simulink model "MLIinverter"  (R2021a)
settings: Solver=FixedStepAuto  StartTime=0.0  StopTime=1  FixedStep=1e-6  RelTol=1e-3
libraries: spsMosfetLib x24, neural x19, spsTriangleGeneratorLib x12, spsSeriesRLCBranchLib x9, spsSeriesRLCLoadLib x4, spsRMSLib x3, spsVoltageMeasurementLib x3, spsThreePhaseVIMeasurementLib x2, spsNeutralLib x1, spsPVArrayLib x1, simulink x1, spsCurrentMeasurementLib x1
(part 1 of 2)
settings Model: Creator=Administrator  LastModifiedBy=dezir
settings SolverCC: AlgebraicLoopSolver=TrustRegion
settings DebuggingCC: SFMachineParentedDataDiag=warning
settings SFSimCC: CustomCodeUndefinedFunction=UseInterfaceOnly

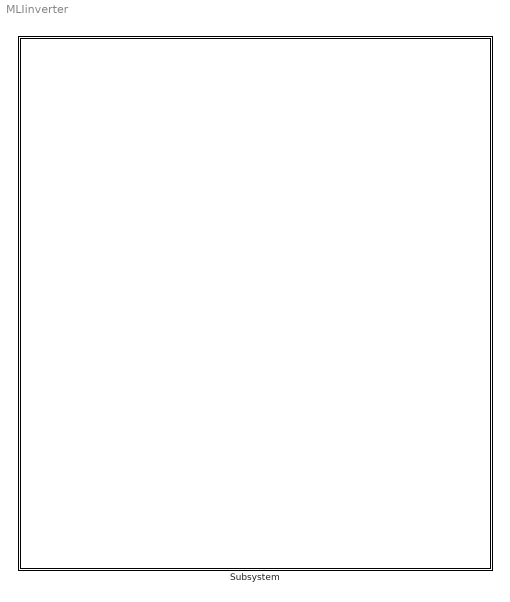
== system MLIinverter ==
  Subsystem : Subsystem

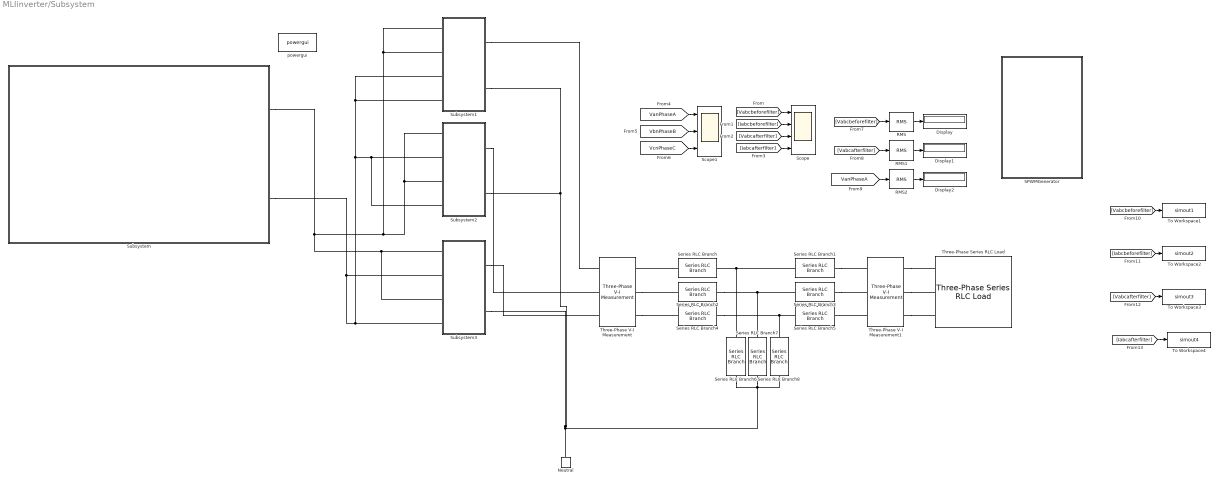
== system MLIinverter/Subsystem ==
  Display : Display
  Display1 : Display
  Display2 : Display
  Neutral : spsNeutralLib/Neutral  LConnTagsString=a  NodeNumber=10
      settings: AttributesFormatString=node %<NodeNumber>  SourceProductBaseCode=PS
  RMS : spsRMSLib/RMS  TrueRMS=on  Freq=50  RMSInit=0  Ts=0
  RMS1 : spsRMSLib/RMS  TrueRMS=on  Freq=50  RMSInit=0  Ts=0
  RMS2 : spsRMSLib/RMS  TrueRMS=on  Freq=50  RMSInit=0  Ts=0
  SPWMGenerator : Subsystem
  Scope : Scope  NumInputPorts=4
  Scope1 : Scope  NumInputPorts=3
  Series RLC Branch : spsSeriesRLCBranchLib/Series RLC Branch  LConnTagsString=__new0  RConnTagsString=__new0  BranchType=L  Resistance=1  Inductance=260e-3  SetiL0=off  InitialCurrent=0  Capacitance=1e-6  Setx0=off  InitialVoltage=0  Measurements=None
  Series RLC Branch1 : spsSeriesRLCBranchLib/Series RLC Branch  LConnTagsString=__new0  RConnTagsString=__new0  BranchType=L  Resistance=1  Inductance=14e-3  SetiL0=off  InitialCurrent=0  Capacitance=1e-6  Setx0=off  InitialVoltage=0  Measurements=None
  Series RLC Branch2 : spsSeriesRLCBranchLib/Series RLC Branch  LConnTagsString=__new0  RConnTagsString=__new0  BranchType=L  Resistance=1  Inductance=260e-3  SetiL0=off  InitialCurrent=0  Capacitance=1e-6  Setx0=off  InitialVoltage=0  Measurements=None
  Series RLC Branch3 : spsSeriesRLCBranchLib/Series RLC Branch  LConnTagsString=__new0  RConnTagsString=__new0  BranchType=L  Resistance=1  Inductance=14e-3  SetiL0=off  InitialCurrent=0  Capacitance=1e-6  Setx0=off  InitialVoltage=0  Measurements=None
  Series RLC Branch4 : spsSeriesRLCBranchLib/Series RLC Branch  LConnTagsString=__new0  RConnTagsString=__new0  BranchType=L  Resistance=1  Inductance=260e-3  SetiL0=off  InitialCurrent=0  Capacitance=1e-6  Setx0=off  InitialVoltage=0  Measurements=None
  Series RLC Branch5 : spsSeriesRLCBranchLib/Series RLC Branch  LConnTagsString=__new0  RConnTagsString=__new0  BranchType=L  Resistance=1  Inductance=14e-3  SetiL0=off  InitialCurrent=0  Capacitance=1e-6  Setx0=off  InitialVoltage=0  Measurements=None
  Series RLC Branch6 : spsSeriesRLCBranchLib/Series RLC Branch  LConnTagsString=__new0  RConnTagsString=__new0  BranchType=C  Resistance=1  Inductance=1e-3  SetiL0=off  InitialCurrent=0  Capacitance=5e-6  Setx0=off  InitialVoltage=0  Measurements=None
  Series RLC Branch7 : spsSeriesRLCBranchLib/Series RLC Branch  LConnTagsString=__new0  RConnTagsString=__new0  BranchType=C  Resistance=1  Inductance=1e-3  SetiL0=off  InitialCurrent=0  Capacitance=5e-6  Setx0=off  InitialVoltage=0  Measurements=None
  Series RLC Branch8 : spsSeriesRLCBranchLib/Series RLC Branch  LConnTagsString=__new0  RConnTagsString=__new0  BranchType=C  Resistance=1  Inductance=1e-3  SetiL0=off  InitialCurrent=0  Capacitance=5e-6  Setx0=off  InitialVoltage=0  Measurements=None
  Subsystem : Subsystem
  Subsystem1 : Subsystem
  Subsystem2 : Subsystem
  Subsystem3 : Subsystem
  Three-Phase Series RLC Load : spsThreePhaseSeriesRLCLoadLib/Three-Phase Series RLC Load  LConnTagsString=A|B|C  Configuration=Y (grounded)  NominalVoltage=400  Vabc=[1e3 1e3 1e3]  Vabcp=[1e3 1e3 1e3]  NominalFrequency=50  UnbalancedPower=off  ActivePower=1e3  InductivePower=0  CapacitivePower=0  Pabc=[10e3 9e3 11e3]  QLabc=[100 90 110]  QCabc=[100 90 110]  Pabcp=[10e3 9e3 11e3]  QLabcp=[100 90 110]  QCabcp=[100 90 110]  Measurements=None  LoadType=constant PQ
  Three-Phase V-I Measurement : spsThreePhaseVIMeasurementLib/Three-Phase V-I Measurement  VoltageMeasurement=phase-to-ground  SetLabelV=on  LabelV=Vabcbeforefilter  Vpu=off  VpuLL=off  CurrentMeasurement=yes  SetLabelI=on  LabelI=Iabcbeforefilter  Ipu=off  Pbase=100e6  Vbase=500e3  OutputType=Complex  PhasorSimulation=off  PSBequivalent=0
  Three-Phase V-I Measurement1 : spsThreePhaseVIMeasurementLib/Three-Phase V-I Measurement  VoltageMeasurement=phase-to-ground  SetLabelV=on  LabelV=Vabcafterfilter  Vpu=off  VpuLL=off  CurrentMeasurement=yes  SetLabelI=on  LabelI=Iabcafterfilter  Ipu=off  Pbase=100e6  Vbase=500e3  OutputType=Complex  PhasorSimulation=off  PSBequivalent=0
  To Workspace1 : ToWorkspace  VariableName=simout1  SaveFormat=Timeseries  SampleTime=-1
  To Workspace2 : ToWorkspace  VariableName=simout2  SaveFormat=Timeseries  SampleTime=-1
  To Workspace3 : ToWorkspace  VariableName=simout3  SaveFormat=Timeseries  SampleTime=-1
  To Workspace4 : ToWorkspace  VariableName=simout4  SaveFormat=Timeseries  SampleTime=-1
  powergui : spspowerguiLib/powergui  Priority=1  SimulationMode=Discrete  SampleTime=6e-6  frequency=60  Iterations=50  frequencyindice=0  Pbase=100e6  ErrMax=1e-4  UnitsV=kV  UnitsW=MW  buscounter=0  FunctionMessages=off  echomessages=off  EnableUseOfTLC=off  CurrentSourceSwitches=off  DisableSnubberDevices=off  DisableRonSwitches=off  DisableVfSwitches=off  DisplayEquations=off  AutomaticDiscreteSolvers=off  SolverType=Tustin/Backward Euler (TBE)  Interpol=off  ExternalGateDelay=off  methode=off  Ts=100  x0status=blocks  SPID=on  SwTol=0  HookPort=off  NonlinearTolerance=0  nMaxIteration=15  ContinueOnMaxIteration=off  RestoreLinks=warning  ResistiveCurrentMeasurement=off  Frange=[0:2:500]  Ylog=off  Xlog=on  ShowGrid=off  save=off  variable=ZData  structure=0  ZoomFFT=off  StartTime=0.0  cycles=1  DisplayStyle=1  fundamental=60  FreqAxis=off  MaxFrequency=1000  frequencyindicesteady=1  RmsSteady=1  display=off
  wires:
  [Iabcbeforefilter] -> Scope/2
  [VcnPhaseC] -> Scope1/3
  [Iabcafterfilter] -> Scope/4
  RMS/1 -> Display/1
  [VanPhaseA] -> Scope1/1
  [VbnPhaseB] -> Scope1/2
  [Vabcbeforefilter] -> Scope/1
  [VanPhaseA] -> RMS2/1
  [Iabcbeforefilter] -> To Workspace2/1
  RMS1/1 -> Display1/1
  [Vabcafterfilter] -> To Workspace3/1
  [Vabcafterfilter] -> RMS1/1
  [Vabcafterfilter] -> Scope/3
  [Iabcafterfilter] -> To Workspace4/1
  RMS2/1 -> Display2/1
  [Vabcbeforefilter] -> RMS/1
  [Vabcbeforefilter] -> To Workspace1/1
  connections:
  Series RLC Branch4/RConn1 -- Series RLC Branch8/LConn1 -- Series RLC Branch5/LConn1
  Series RLC Branch/LConn1 -- Three-Phase V-I Measurement/RConn1
  Three-Phase V-I Measurement/RConn2 -- Series RLC Branch2/LConn1
  Series RLC Branch2/RConn1 -- Series RLC Branch7/LConn1 -- Series RLC Branch3/LConn1
  Series RLC Branch3/RConn1 -- Three-Phase V-I Measurement1/LConn2
  Series RLC Branch1/LConn1 -- Series RLC Branch6/LConn1 -- Series RLC Branch/RConn1
  Three-Phase V-I Measurement1/RConn1 -- Three-Phase Series RLC Load/LConn1
  Subsystem2/RConn2 -- Subsystem1/RConn2 -- Subsystem3/RConn2 -- Neutral/LConn1 -- Series RLC Branch7/RConn1 -- Series RLC Branch6/RConn1 -- Series RLC Branch8/RConn1
  Three-Phase V-I Measurement1/LConn3 -- Series RLC Branch5/RConn1
  Three-Phase V-I Measurement/RConn3 -- Series RLC Branch4/LConn1
  Three-Phase V-I Measurement1/RConn3 -- Three-Phase Series RLC Load/LConn3
  Series RLC Branch1/RConn1 -- Three-Phase V-I Measurement1/LConn1
  Three-Phase V-I Measurement1/RConn2 -- Three-Phase Series RLC Load/LConn2
  Subsystem1/RConn1 -- Three-Phase V-I Measurement/LConn1
  Subsystem/RConn1 -- Subsystem3/LConn3 -- Subsystem3/LConn1 -- Subsystem2/LConn1 -- Subsystem2/LConn3 -- Subsystem1/LConn1 -- Subsystem1/LConn2
  Subsystem/RConn2 -- Subsystem3/LConn4 -- Subsystem2/LConn2 -- Subsystem2/LConn4 -- Subsystem1/LConn4 -- Subsystem1/LConn3 -- Subsystem3/LConn2
  Subsystem2/RConn1 -- Three-Phase V-I Measurement/LConn2
  Subsystem3/RConn1 -- Three-Phase V-I Measurement/LConn3

== system MLIinverter/Subsystem/SPWMGenerator ==
  spwmGen : Subsystem
  spwmGen1 : Subsystem
  spwmGen2 : Subsystem

== system MLIinverter/Subsystem/Subsystem ==
  Custom Neural Network : Subsystem
      mask help: Custom Neural Network
      mask Display: e = 0.06;c1 = [120 150 230]/255;c2 = ([120 150 230]+0)/383;c3 = ([120 150 230]+128)/383;patch([0 1 1 0],[0 0 1 1],c1);patch([0 1 1 1-e 1-e 0+e],[0 0 1 1-e 0+e 0+e],c2);patch([0 0 1 1-e 0+e 0+e],[0 1 1 1-e 1-e 0+e],c3);plot([0 1 1 0 0],[0 0 1 1 0]);fprintf('NNET');port_label('input',1,' Input');port_label('output',1,'Output ');
  PV Array : spsPVArrayLib/PV Array  Npar=20  Nser=10  PlotType=array @ 25 deg.C & specified irradiances  S_vec="[ 1000  500  100 ]"  Temp_C_vec="[ 45 25  ]"  ModuleName=A10Green Technology A10J-M60-240  PlotWhenSelected=off  Pm=240.5376  Ncell=60  Voc=36.84  Isc=8.32  Vm=30.72  Im=7.83  beta_Voc_pc=-0.359  alpha_Isc_pc=0.096995  beta_Voc=-0.13226  alpha_Isc=0.00807  IL=8.3299  I0=2.8736e-10  nI=0.99259  Rsh=330.6558  Rs=0.19366  RobustModel=off  RobustCellTemperature=313.3991  BAL=on  Tc=1e-6  Tfilter=5e-5
  Repeating Sequence : simulink/Sources/Repeating Sequence  rep_seq_t=[0 100]  rep_seq_y=[15 40]
  Subsystem1 : Subsystem
  Subsystem2 : Subsystem
  Uniform Random Number : UniformRandomNumber  Minimum=800  Maximum=1000  SampleTime=0.1
  D : PMIOPort  Side=Right
  S : PMIOPort  Port=2  Side=Right
  tag scope: Irr=global, temp=global
  wires:
  PV Array/1 -> Subsystem1/2(In2)
  Uniform Random Number/1 -> [Irr], PV Array/1
  Repeating Sequence/1 -> [temp], PV Array/2
  Subsystem1/1(Out1) -> Custom Neural Network/1(Input)
  Custom Neural Network/1(Output) -> Subsystem1/1(In1)
  connections:
  Subsystem1/RConn5 -- S/RConn1 -- Subsystem1/RConn4 -- PV Array/RConn2 -- Subsystem1/RConn2 -- Subsystem1/RConn3
  PV Array/RConn1 -- Subsystem1/LConn1
  D/RConn1 -- Subsystem1/RConn1

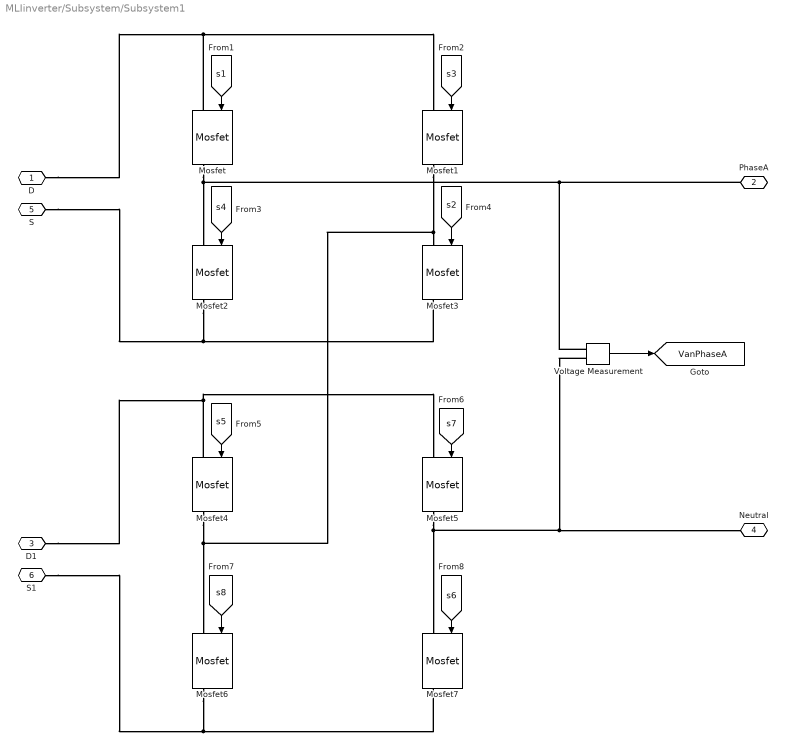
== system MLIinverter/Subsystem/Subsystem1 ==
  Mosfet{,1..7} (8 alike) : spsMosfetLib/Mosfet  Ron=0.1  Lon=0  Rd=0.01  Vfd=0  IC=0  Rs=1e5  Cs=inf  Measurements=on
  Voltage Measurement : spsVoltageMeasurementLib/Voltage Measurement  PhasorSimulation=off  OutputType=Complex  PSBequivalent=0
  D : PMIOPort  Side=Left
  PhaseA : PMIOPort  Port=2  Side=Right
  D1 : PMIOPort  Port=3  Side=Left
  Neutral : PMIOPort  Port=4  Side=Right
  S : PMIOPort  Port=5  Side=Left
  S1 : PMIOPort  Port=6  Side=Left
  tag scope: VanPhaseA=global
  wires:
  [s7] -> Mosfet5/1
  [s4] -> Mosfet2/1
  [s8] -> Mosfet6/1
  [s6] -> Mosfet7/1
  [s2] -> Mosfet3/1
  Voltage Measurement/1 -> [VanPhaseA]
  [s5] -> Mosfet4/1
  [s3] -> Mosfet1/1
  [s1] -> Mosfet/1
  connections:
  Voltage Measurement/LConn1 -- Mosfet/RConn1 -- Mosfet2/LConn1 -- PhaseA/RConn1
  Mosfet/LConn1 -- Mosfet1/LConn1 -- D/RConn1
  D1/RConn1 -- Mosfet4/LConn1 -- Mosfet5/LConn1
  Voltage Measurement/LConn2 -- Mosfet5/RConn1 -- Mosfet7/LConn1 -- Neutral/RConn1
  Mosfet6/RConn1 -- Mosfet7/RConn1 -- S1/RConn1
  Mosfet1/RConn1 -- Mosfet4/RConn1 -- Mosfet6/LConn1 -- Mosfet3/LConn1
  Mosfet2/RConn1 -- Mosfet3/RConn1 -- S/RConn1

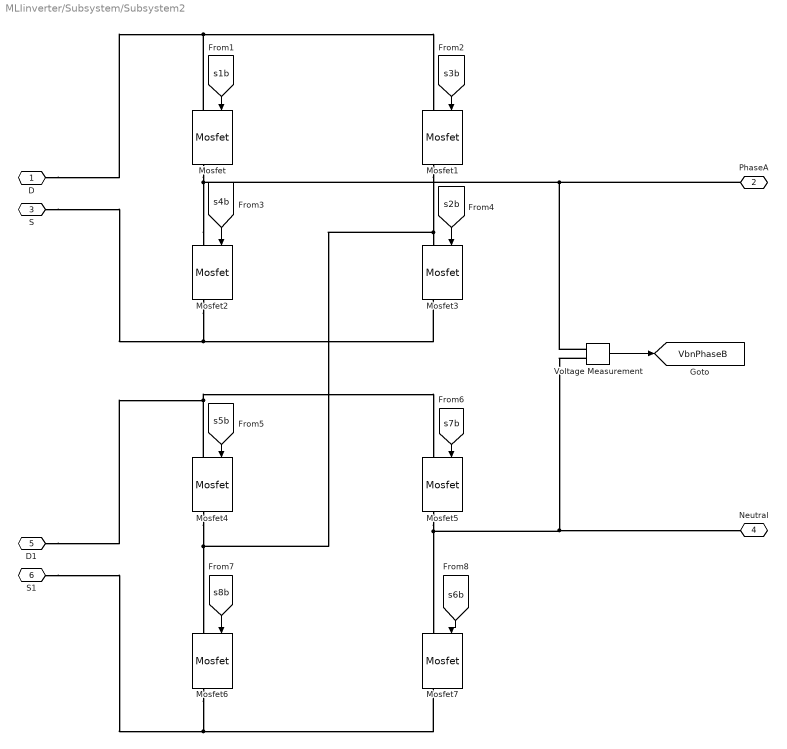
== system MLIinverter/Subsystem/Subsystem2 ==
  Mosfet{,1..7} (8 alike) : spsMosfetLib/Mosfet  Ron=0.1  Lon=0  Rd=0.01  Vfd=0  IC=0  Rs=1e5  Cs=inf  Measurements=on
  Voltage Measurement : spsVoltageMeasurementLib/Voltage Measurement  PhasorSimulation=off  OutputType=Complex  PSBequivalent=0
  D : PMIOPort  Side=Left
  PhaseA : PMIOPort  Port=2  Side=Right
  S : PMIOPort  Port=3  Side=Left
  Neutral : PMIOPort  Port=4  Side=Right
  D1 : PMIOPort  Port=5  Side=Left
  S1 : PMIOPort  Port=6  Side=Left
  tag scope: VbnPhaseB=global
  wires:
  [s7b] -> Mosfet5/1
  [s8b] -> Mosfet6/1
  [s5b] -> Mosfet4/1
  [s2b] -> Mosfet3/1
  [s3b] -> Mosfet1/1
  [s6b] -> Mosfet7/1
  [s1b] -> Mosfet/1
  [s4b] -> Mosfet2/1
  Voltage Measurement/1 -> [VbnPhaseB]
  connections:
  Voltage Measurement/LConn2 -- Mosfet7/LConn1 -- Mosfet5/RConn1 -- Neutral/RConn1
  D1/RConn1 -- Mosfet4/LConn1 -- Mosfet5/LConn1
  Mosfet/LConn1 -- Mosfet1/LConn1 -- D/RConn1
  Mosfet1/RConn1 -- Mosfet6/LConn1 -- Mosfet4/RConn1 -- Mosfet3/LConn1
  Mosfet7/RConn1 -- Mosfet6/RConn1 -- S1/RConn1
  Mosfet2/RConn1 -- Mosfet3/RConn1 -- S/RConn1
  Mosfet2/LConn1 -- Mosfet/RConn1 -- Voltage Measurement/LConn1 -- PhaseA/RConn1

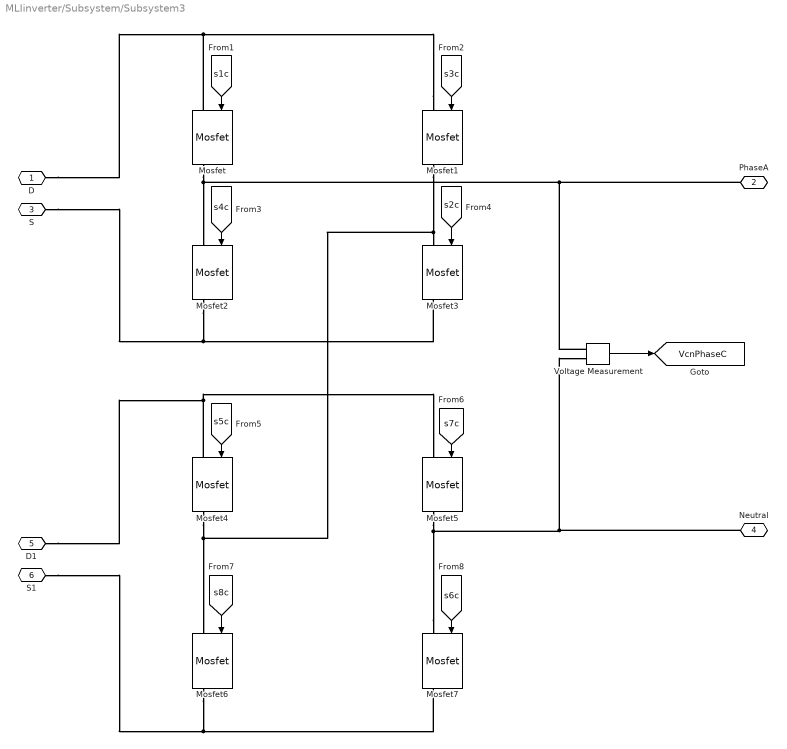
== system MLIinverter/Subsystem/Subsystem3 ==
  Mosfet{,1..7} (8 alike) : spsMosfetLib/Mosfet  Ron=0.1  Lon=0  Rd=0.01  Vfd=0  IC=0  Rs=1e5  Cs=inf  Measurements=on
  Voltage Measurement : spsVoltageMeasurementLib/Voltage Measurement  PhasorSimulation=off  OutputType=Complex  PSBequivalent=0
  D : PMIOPort  Side=Left
  PhaseA : PMIOPort  Port=2  Side=Right
  S : PMIOPort  Port=3  Side=Left
  Neutral : PMIOPort  Port=4  Side=Right
  D1 : PMIOPort  Port=5  Side=Left
  S1 : PMIOPort  Port=6  Side=Left
  tag scope: VcnPhaseC=global
  wires:
  [s2c] -> Mosfet3/1
  [s4c] -> Mosfet2/1
  [s6c] -> Mosfet7/1
  [s1c] -> Mosfet/1
  [s3c] -> Mosfet1/1
  Voltage Measurement/1 -> [VcnPhaseC]
  [s7c] -> Mosfet5/1
  [s8c] -> Mosfet6/1
  [s5c] -> Mosfet4/1
  connections:
  Mosfet6/RConn1 -- Mosfet7/RConn1 -- S1/RConn1
  Voltage Measurement/LConn1 -- Mosfet/RConn1 -- Mosfet2/LConn1 -- PhaseA/RConn1
  Mosfet7/LConn1 -- Mosfet5/RConn1 -- Voltage Measurement/LConn2 -- Neutral/RConn1
  Mosfet1/LConn1 -- Mosfet/LConn1 -- D/RConn1
  D1/RConn1 -- Mosfet4/LConn1 -- Mosfet5/LConn1
  Mosfet1/RConn1 -- Mosfet6/LConn1 -- Mosfet4/RConn1 -- Mosfet3/LConn1
  Mosfet3/RConn1 -- Mosfet2/RConn1 -- S/RConn1

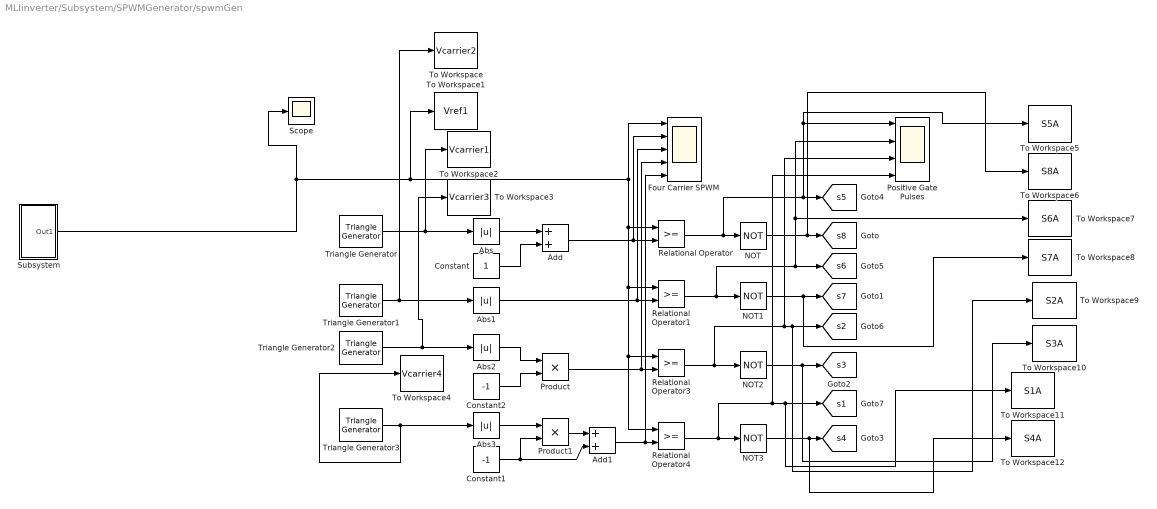
== system MLIinverter/Subsystem/SPWMGenerator/spwmGen ==
  Abs{,1..3} (4 alike) : Abs
  Add : Sum
  Add1 : Sum
  Constant : Constant
  Constant1 : Constant  Value=-1
  Constant2 : Constant  Value=-1
  Four Carrier SPWM : Scope  NumInputPorts=5
  NOT{,1..3} (4 alike) : Logic  Operator=NOT  IconShape=distinctive  AllPortsSameDT=off  OutDataTypeStr=boolean
  Positive Gate Pulses : Scope  NumInputPorts=4
  Product : Product
  Product1 : Product
  Relational Operator{,1,3..4} (4 alike) : RelationalOperator  OutDataTypeStr=boolean  RndMeth=Simplest
  Scope : Scope
  Subsystem : Subsystem
  To Workspace : ToWorkspace  VariableName=Vcarrier2  SampleTime=-1
      settings: Save2DSignal=2-D array (concatenate along first dimension)
  To Workspace1 : ToWorkspace  VariableName=Vref1  SampleTime=-1
      settings: Save2DSignal=2-D array (concatenate along first dimension)
  To Workspace10 : ToWorkspace  VariableName=S3A  SaveFormat=Timeseries  SampleTime=-1
      settings: Save2DSignal=2-D array (concatenate along first dimension)
  To Workspace11 : ToWorkspace  VariableName=S1A  SaveFormat=Timeseries  SampleTime=-1
      settings: Save2DSignal=2-D array (concatenate along first dimension)
  To Workspace12 : ToWorkspace  VariableName=S4A  SaveFormat=Timeseries  SampleTime=-1
      settings: Save2DSignal=2-D array (concatenate along first dimension)
  To Workspace2 : ToWorkspace  VariableName=Vcarrier1  SampleTime=-1
      settings: Save2DSignal=2-D array (concatenate along first dimension)
  To Workspace3 : ToWorkspace  VariableName=Vcarrier3  SampleTime=-1
      settings: Save2DSignal=2-D array (concatenate along first dimension)
  To Workspace4 : ToWorkspace  VariableName=Vcarrier4  SampleTime=-1
      settings: Save2DSignal=2-D array (concatenate along first dimension)
  To Workspace5 : ToWorkspace  VariableName=S5A  SaveFormat=Timeseries  SampleTime=-1
      settings: Save2DSignal=2-D array (concatenate along first dimension)
  To Workspace6 : ToWorkspace  VariableName=S8A  SaveFormat=Timeseries  SampleTime=-1
      settings: Save2DSignal=2-D array (concatenate along first dimension)
  To Workspace7 : ToWorkspace  VariableName=S6A  SaveFormat=Timeseries  SampleTime=-1
      settings: Save2DSignal=2-D array (concatenate along first dimension)
  To Workspace8 : ToWorkspace  VariableName=S7A  SaveFormat=Timeseries  SampleTime=-1
      settings: Save2DSignal=2-D array (concatenate along first dimension)
  To Workspace9 : ToWorkspace  VariableName=S2A  SaveFormat=Timeseries  SampleTime=-1
      settings: Save2DSignal=2-D array (concatenate along first dimension)
  Triangle Generator : spsTriangleGeneratorLib/Triangle Generator  Freq=10e3  Phase=90  Ts=0
  Triangle Generator1 : spsTriangleGeneratorLib/Triangle Generator  Freq=10e3  Phase=90  Ts=0
  Triangle Generator2 : spsTriangleGeneratorLib/Triangle Generator  Freq=10e3  Phase=0  Ts=0
  Triangle Generator3 : spsTriangleGeneratorLib/Triangle Generator  Freq=10e3  Phase=0  Ts=0
  tag scope: s1=global, s2=global, s3=global, s4=global, s5=global, s6=global, s7=global, s8=global
  wires:
  Product1/1 -> Add1/1
  Add1/1 -> Four Carrier SPWM/5, Relational Operator4/2
  NOT3/1 -> To Workspace12/1, [s4]
  Subsystem/1(Out1) -> Scope/1, To Workspace1/1, Four Carrier SPWM/1, Relational Operator/1, Relational Operator4/1, Relational Operator3/1, Relational Operator1/1
  Triangle Generator/1 -> To Workspace2/1, Abs/1
  Constant1/1 -> Add1/2, Product1/2
  Relational Operator/1 -> To Workspace5/1, Positive Gate Pulses/1, [s5], NOT/1
  Add/1 -> Relational Operator/2, Four Carrier SPWM/2
  NOT/1 -> To Workspace6/1, [s8]
  Abs3/1 -> Product1/1
  Abs/1 -> Add/1
  NOT1/1 -> To Workspace8/1, [s7]
  Relational Operator3/1 -> Positive Gate Pulses/3, To Workspace9/1, [s2], NOT2/1
  Abs1/1 -> Relational Operator1/2, Four Carrier SPWM/3
  NOT2/1 -> To Workspace10/1, [s3]
  Product/1 -> Relational Operator3/2, Four Carrier SPWM/4
  Relational Operator1/1 -> To Workspace7/1, Positive Gate Pulses/2, [s6], NOT1/1
  Relational Operator4/1 -> Positive Gate Pulses/4, To Workspace11/1, [s1], NOT3/1
  Triangle Generator3/1 -> To Workspace4/1, Abs3/1
  Triangle Generator1/1 -> To Workspace/1, Abs1/1
  Constant/1 -> Add/2
  Triangle Generator2/1 -> To Workspace3/1, Abs2/1
  Abs2/1 -> Product/1
  Constant2/1 -> Product/2

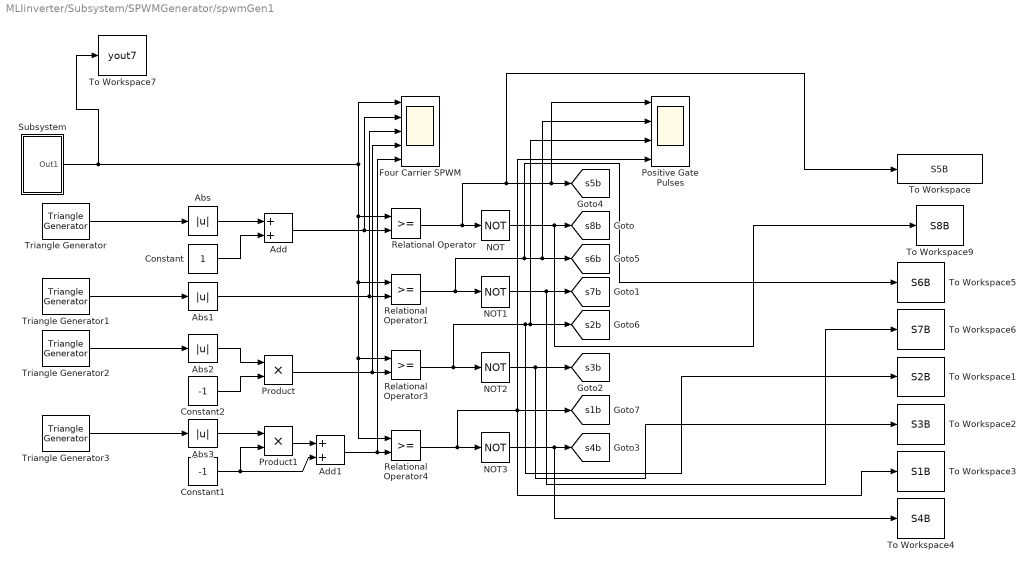
== system MLIinverter/Subsystem/SPWMGenerator/spwmGen1 ==
  Abs{,1..3} (4 alike) : Abs
  Add : Sum
  Add1 : Sum
  Constant : Constant
  Constant1 : Constant  Value=-1
  Constant2 : Constant  Value=-1
  Four Carrier SPWM : Scope  NumInputPorts=5
  NOT{,1..3} (4 alike) : Logic  Operator=NOT  IconShape=distinctive  AllPortsSameDT=off  OutDataTypeStr=boolean
  Positive Gate Pulses : Scope  NumInputPorts=4
  Product : Product
  Product1 : Product
  Relational Operator{,1,3..4} (4 alike) : RelationalOperator  OutDataTypeStr=boolean  RndMeth=Simplest
  Subsystem : Subsystem
  To Workspace : ToWorkspace  VariableName=S5B  SaveFormat=Timeseries  SampleTime=-1
      settings: Save2DSignal=2-D array (concatenate along first dimension)
  To Workspace1 : ToWorkspace  VariableName=S2B  SaveFormat=Timeseries  SampleTime=-1
      settings: Save2DSignal=2-D array (concatenate along first dimension)
  To Workspace2 : ToWorkspace  VariableName=S3B  SaveFormat=Timeseries  SampleTime=-1
      settings: Save2DSignal=2-D array (concatenate along first dimension)
  To Workspace3 : ToWorkspace  VariableName=S1B  SaveFormat=Timeseries  SampleTime=-1
      settings: Save2DSignal=2-D array (concatenate along first dimension)
  To Workspace4 : ToWorkspace  VariableName=S4B  SaveFormat=Timeseries  SampleTime=-1
      settings: Save2DSignal=2-D array (concatenate along first dimension)
  To Workspace5 : ToWorkspace  VariableName=S6B  SaveFormat=Timeseries  SampleTime=-1
      settings: Save2DSignal=2-D array (concatenate along first dimension)
  To Workspace6 : ToWorkspace  VariableName=S7B  SaveFormat=Timeseries  SampleTime=-1
      settings: Save2DSignal=2-D array (concatenate along first dimension)
  To Workspace7 : ToWorkspace  VariableName=yout7  SampleTime=-1
      settings: Save2DSignal=2-D array (concatenate along first dimension)
  To Workspace9 : ToWorkspace  VariableName=S8B  SaveFormat=Timeseries  SampleTime=-1
      settings: Save2DSignal=2-D array (concatenate along first dimension)
  Triangle Generator : spsTriangleGeneratorLib/Triangle Generator  Freq=10e3  Phase=90  Ts=0
  Triangle Generator1 : spsTriangleGeneratorLib/Triangle Generator  Freq=10e3  Phase=90  Ts=0
  Triangle Generator2 : spsTriangleGeneratorLib/Triangle Generator  Freq=10e3  Phase=0  Ts=0
  Triangle Generator3 : spsTriangleGeneratorLib/Triangle Generator  Freq=10e3  Phase=0  Ts=0
  tag scope: s1b=global, s2b=global, s3b=global, s4b=global, s5b=global, s6b=global, s7b=global, s8b=global
  wires:
  Constant2/1 -> Product/2
  Abs2/1 -> Product/1
  Triangle Generator2/1 -> Abs2/1
  Constant/1 -> Add/2
  Triangle Generator1/1 -> Abs1/1
  Triangle Generator3/1 -> Abs3/1
  Relational Operator4/1 -> NOT3/1, To Workspace3/1, [s1b], Positive Gate Pulses/4
  Relational Operator1/1 -> NOT1/1, To Workspace5/1, [s6b], Positive Gate Pulses/2
  Product/1 -> Four Carrier SPWM/4, Relational Operator3/2
  NOT2/1 -> To Workspace2/1, [s3b]
  Abs1/1 -> Four Carrier SPWM/3, Relational Operator1/2
  Relational Operator3/1 -> NOT2/1, To Workspace1/1, [s2b], Positive Gate Pulses/3
  NOT1/1 -> To Workspace6/1, [s7b]
  Abs/1 -> Add/1
  Abs3/1 -> Product1/1
  NOT/1 -> To Workspace9/1, [s8b]
  Add/1 -> Four Carrier SPWM/2, Relational Operator/2
  Relational Operator/1 -> NOT/1, To Workspace/1, [s5b], Positive Gate Pulses/1
  Constant1/1 -> Product1/2, Add1/2
  Triangle Generator/1 -> Abs/1
  Subsystem/1(Out1) -> To Workspace7/1, Relational Operator1/1, Relational Operator3/1, Relational Operator4/1, Relational Operator/1, Four Carrier SPWM/1
  NOT3/1 -> To Workspace4/1, [s4b]
  Add1/1 -> Relational Operator4/2, Four Carrier SPWM/5
  Product1/1 -> Add1/1

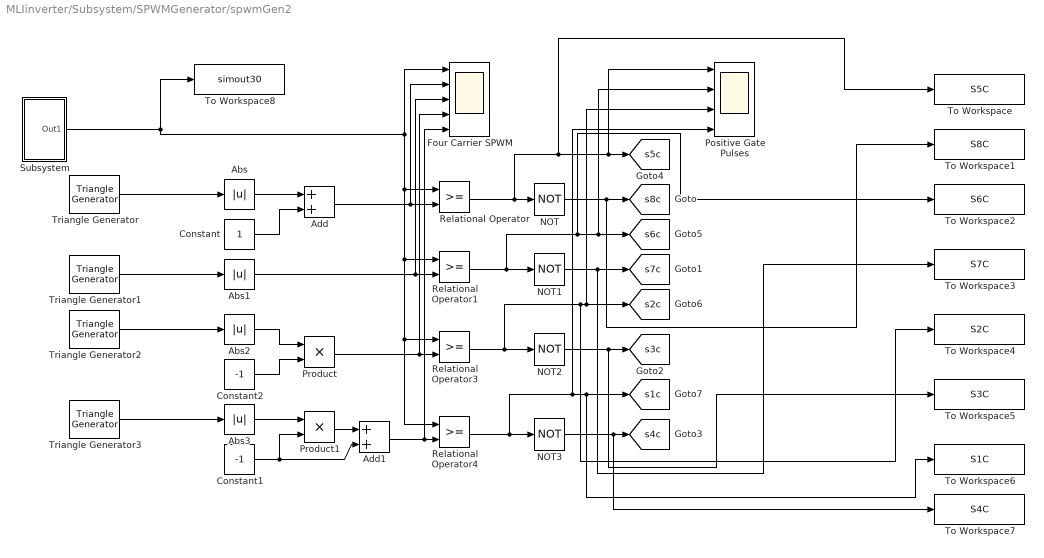
== system MLIinverter/Subsystem/SPWMGenerator/spwmGen2 ==
  Abs{,1..3} (4 alike) : Abs
  Add : Sum
  Add1 : Sum
  Constant : Constant
  Constant1 : Constant  Value=-1
  Constant2 : Constant  Value=-1
  Four Carrier SPWM : Scope  NumInputPorts=5
  NOT{,1..3} (4 alike) : Logic  Operator=NOT  IconShape=distinctive  AllPortsSameDT=off  OutDataTypeStr=boolean
  Positive Gate Pulses : Scope  NumInputPorts=4
  Product : Product
  Product1 : Product
  Relational Operator{,1,3..4} (4 alike) : RelationalOperator  OutDataTypeStr=boolean  RndMeth=Simplest
  Subsystem : Subsystem
  To Workspace : ToWorkspace  VariableName=S5C  SaveFormat=Timeseries  SampleTime=-1
      settings: Save2DSignal=2-D array (concatenate along first dimension)
  To Workspace1 : ToWorkspace  VariableName=S8C  SaveFormat=Timeseries  SampleTime=-1
      settings: Save2DSignal=2-D array (concatenate along first dimension)
  To Workspace2 : ToWorkspace  VariableName=S6C  SaveFormat=Timeseries  SampleTime=-1
      settings: Save2DSignal=2-D array (concatenate along first dimension)
  To Workspace3 : ToWorkspace  VariableName=S7C  SaveFormat=Timeseries  SampleTime=-1
      settings: Save2DSignal=2-D array (concatenate along first dimension)
  To Workspace4 : ToWorkspace  VariableName=S2C  SaveFormat=Timeseries  SampleTime=-1
      settings: Save2DSignal=2-D array (concatenate along first dimension)
  To Workspace5 : ToWorkspace  VariableName=S3C  SaveFormat=Timeseries  SampleTime=-1
      settings: Save2DSignal=2-D array (concatenate along first dimension)
  To Workspace6 : ToWorkspace  VariableName=S1C  SaveFormat=Timeseries  SampleTime=-1
      settings: Save2DSignal=2-D array (concatenate along first dimension)
  To Workspace7 : ToWorkspace  VariableName=S4C  SaveFormat=Timeseries  SampleTime=-1
      settings: Save2DSignal=2-D array (concatenate along first dimension)
  To Workspace8 : ToWorkspace  VariableName=simout30  SampleTime=-1
      settings: Save2DSignal=2-D array (concatenate along first dimension)
  Triangle Generator : spsTriangleGeneratorLib/Triangle Generator  Freq=10e3  Phase=90  Ts=0
  Triangle Generator1 : spsTriangleGeneratorLib/Triangle Generator  Freq=10e3  Phase=90  Ts=0
  Triangle Generator2 : spsTriangleGeneratorLib/Triangle Generator  Freq=10e3  Phase=0  Ts=0
  Triangle Generator3 : spsTriangleGeneratorLib/Triangle Generator  Freq=10e3  Phase=0  Ts=0
  tag scope: s1c=global, s2c=global, s3c=global, s4c=global, s5c=global, s6c=global, s7c=global, s8c=global
  wires:
  Product1/1 -> Add1/1
  Add1/1 -> Four Carrier SPWM/5, Relational Operator4/2
  NOT3/1 -> To Workspace7/1, [s4c]
  Subsystem/1(Out1) -> Four Carrier SPWM/1, Relational Operator/1, Relational Operator4/1, Relational Operator3/1, Relational Operator1/1, To Workspace8/1
  Triangle Generator/1 -> Abs/1
  Constant1/1 -> Add1/2, Product1/2
  Relational Operator/1 -> To Workspace/1, Positive Gate Pulses/1, [s5c], NOT/1
  Add/1 -> Relational Operator/2, Four Carrier SPWM/2
  NOT/1 -> To Workspace1/1, [s8c]
  Abs3/1 -> Product1/1
  Abs/1 -> Add/1
  NOT1/1 -> To Workspace3/1, [s7c]
  Relational Operator3/1 -> To Workspace4/1, Positive Gate Pulses/3, [s2c], NOT2/1
  Abs1/1 -> Relational Operator1/2, Four Carrier SPWM/3
  NOT2/1 -> To Workspace5/1, [s3c]
  Product/1 -> Relational Operator3/2, Four Carrier SPWM/4
  Relational Operator1/1 -> To Workspace2/1, Positive Gate Pulses/2, [s6c], NOT1/1
  Relational Operator4/1 -> Positive Gate Pulses/4, To Workspace6/1, [s1c], NOT3/1
  Triangle Generator3/1 -> Abs3/1
  Triangle Generator1/1 -> Abs1/1
  Constant/1 -> Add/2
  Triangle Generator2/1 -> Abs2/1
  Abs2/1 -> Product/1
  Constant2/1 -> Product/2

== system MLIinverter/Subsystem/Subsystem/Custom Neural Network ==
  Input : Inport  PortDimensions=3
      mask Display: e = 0.06;c1 = [120 230 180]/255;c2 = ([120 230 180]+0)/(256+128);c3 = ([120 230 180]+128)/(256+128);patch([0 1 1 0],[0 0 1 1],c1);patch([0 1 1 1-e 1-e 0+e],[0 0 1 1-e 0+e 0+e],c2);patch([0 0 1 1-e 0+e 0+e],[0 1 1 1-e 1-e 0+e],c3);plot([0 1 1 0 0],[0 0 1 1 0]);
  Layer 1 : Subsystem
      mask Display: e = 0.06;c1 = [120 150 230]/255;c2 = ([120 150 230]+0)/383;c3 = ([120 150 230]+128)/383;patch([0 1 1 0],[0 0 1 1],c1);patch([0 1 1 1-e 1-e 0+e],[0 0 1 1-e 0+e 0+e],c2);patch([0 0 1 1-e 0+e 0+e],[0 1 1 1-e 1-e 0+e],c3);plot([0 1 1 0 0],[0 0 1 1 0]);
  Layer 2 : Subsystem
      mask Display: e = 0.06;c1 = [120 150 230]/255;c2 = ([120 150 230]+0)/383;c3 = ([120 150 230]+128)/383;patch([0 1 1 0],[0 0 1 1],c1);patch([0 1 1 1-e 1-e 0+e],[0 0 1 1-e 0+e 0+e],c2);patch([0 0 1 1-e 0+e 0+e],[0 1 1 1-e 1-e 0+e],c3);plot([0 1 1 0 0],[0 0 1 1 0]);
  Layer 3 : Subsystem
      mask Display: e = 0.06;c1 = [120 150 230]/255;c2 = ([120 150 230]+0)/383;c3 = ([120 150 230]+128)/383;patch([0 1 1 0],[0 0 1 1],c1);patch([0 1 1 1-e 1-e 0+e],[0 0 1 1-e 0+e 0+e],c2);patch([0 0 1 1-e 0+e 0+e],[0 1 1 1-e 1-e 0+e],c3);plot([0 1 1 0 0],[0 0 1 1 0]);
  Process Input 1 : Subsystem
      mask Display: e = 0.06;c1 = [120 150 230]/255;c2 = ([120 150 230]+0)/383;c3 = ([120 150 230]+128)/383;patch([0 1 1 0],[0 0 1 1],c1);patch([0 1 1 1-e 1-e 0+e],[0 0 1 1-e 0+e 0+e],c2);patch([0 0 1 1-e 0+e 0+e],[0 1 1 1-e 1-e 0+e],c3);plot([0 1 1 0 0],[0 0 1 1 0]);
  Process Output 1 : Subsystem
      mask Display: e = 0.06;c1 = [120 150 230]/255;c2 = ([120 150 230]+0)/383;c3 = ([120 150 230]+128)/383;patch([0 1 1 0],[0 0 1 1],c1);patch([0 1 1 1-e 1-e 0+e],[0 0 1 1-e 0+e 0+e],c2);patch([0 0 1 1-e 0+e 0+e],[0 1 1 1-e 1-e 0+e],c3);plot([0 1 1 0 0],[0 0 1 1 0]);
  Output : Outport  InitialOutput=0
      mask Display: e = 0.06;c1 = [120 230 180]/255;c2 = ([120 230 180]+0)/(256+128);c3 = ([120 230 180]+128)/(256+128);patch([0 1 1 0],[0 0 1 1],c1);patch([0 1 1 1-e 1-e 0+e],[0 0 1 1-e 0+e 0+e],c2);patch([0 0 1 1-e 0+e 0+e],[0 1 1 1-e 1-e 0+e],c3);plot([0 1 1 0 0],[0 0 1 1 0]);
  wires:
  Input/1 -> Process Input 1/1(x)
  Process Output 1/1(y) -> Output/1
  Process Input 1/1(p) -> Layer 1/1("p{1}")
  Layer 1/1("a{1}") -> [feedback1]
  [feedback1] -> Layer 2/1("a{1} ")
  Layer 2/1("a{2}") -> [feedback2]
  [feedback2] -> Layer 3/1("a{2} ")
  Layer 3/1("a{3}") -> Process Output 1/1(a)

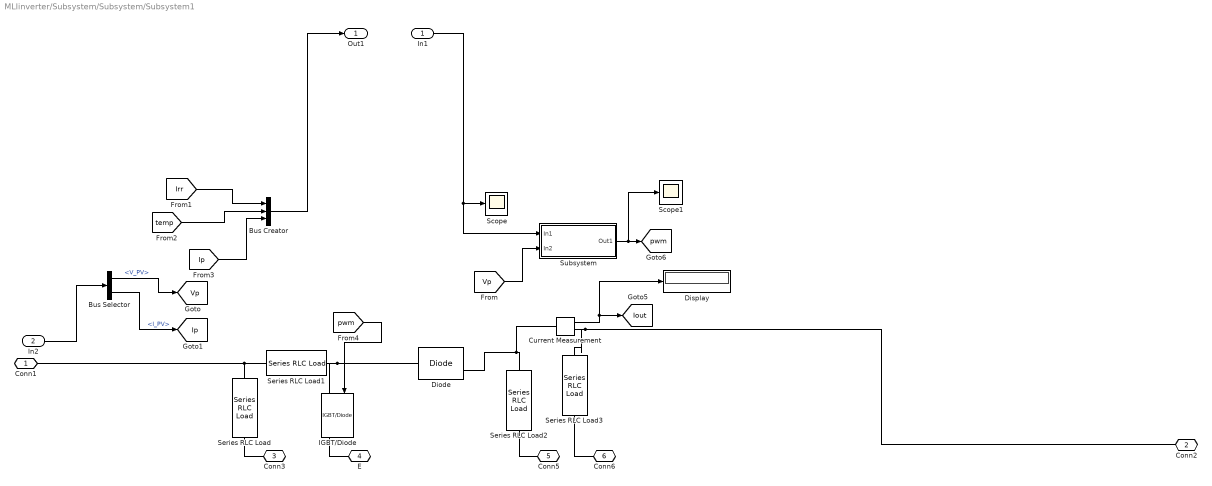
== system MLIinverter/Subsystem/Subsystem/Subsystem1 ==
  In1 : Inport
  In2 : Inport  Port=2
  Bus Creator : BusCreator  Inputs=3
  Bus Selector : BusSelector  OutputSignals=V_PV,I_PV
  Current Measurement : spsCurrentMeasurementLib/Current Measurement  PhasorSimulation=off  OutputType=Complex  PSBequivalent=0
  Diode : spsDiodeLib/Diode  Ron=0.001  Lon=0  Vf=0.8  IC=0  UseSnubber=0  Rs=500  Cs=250e-9  Measurements=on
  Display : Display
  IGBT/Diode : spsIGBTDiodeLib/IGBT//Diode  Ron=1e-3  Rs=1e5  Cs=inf  Measurements=on
  Scope : Scope
  Scope1 : Scope
  Series RLC Load : spsSeriesRLCLoadLib/Series RLC Load  LConnTagsString=a  RConnTagsString=__new0  NominalVoltage=100  NominalFrequency=50  ActivePower=2  InductivePower=0  CapacitivePower=314  Setx0=off  InitialVoltage=0  SetiL0=off  InitialCurrent=0  Measurements=None  LoadType=constant Z
  Series RLC Load1 : spsSeriesRLCLoadLib/Series RLC Load  LConnTagsString=a  RConnTagsString=__new0  NominalVoltage=100  NominalFrequency=50  ActivePower=2  InductivePower=314  CapacitivePower=0  Setx0=off  InitialVoltage=0  SetiL0=off  InitialCurrent=0  Measurements=None  LoadType=constant Z
  Series RLC Load2 : spsSeriesRLCLoadLib/Series RLC Load  LConnTagsString=a  RConnTagsString=__new0  NominalVoltage=100  NominalFrequency=50  ActivePower=2  InductivePower=0  CapacitivePower=314  Setx0=off  InitialVoltage=0  SetiL0=off  InitialCurrent=0  Measurements=None  LoadType=constant Z
  Series RLC Load3 : spsSeriesRLCLoadLib/Series RLC Load  LConnTagsString=a  RConnTagsString=__new0  NominalVoltage=100  NominalFrequency=50  ActivePower=1086.95  InductivePower=0  CapacitivePower=0  Setx0=off  InitialVoltage=0  SetiL0=off  InitialCurrent=0  Measurements=None  LoadType=constant Z
  Subsystem : Subsystem
  Conn1 : PMIOPort  Side=Left
  Conn2 : PMIOPort  Port=2  Side=Right
  Conn3 : PMIOPort  Port=3  Side=Right
  E : PMIOPort  Port=4  Side=Right
  Conn5 : PMIOPort  Port=5  Side=Right
  Conn6 : PMIOPort  Port=6  Side=Right
  Out1 : Outport
  tag scope: Iout=global, Ip=global, Vp=global, pwm=global
  wires:
  In1/1 -> Subsystem/1(In1), Scope/1
  Subsystem/1(Out1) -> Scope1/1, [pwm]
  [temp] -> Bus Creator/2
  [Vp] -> Subsystem/2(In2)
  Bus Selector/2 -> [Ip]  "<I_PV>"
  [pwm] -> IGBT/Diode/1
  [Irr] -> Bus Creator/1
  Bus Selector/1 -> [Vp]  "<V_PV>"
  [Ip] -> Bus Creator/3
  Current Measurement/1 -> Display/1, [Iout]
  In2/1 -> Bus Selector/1
  Bus Creator/1 -> Out1/1
  connections:
  Series RLC Load1/RConn1 -- IGBT/Diode/LConn1 -- Diode/LConn1
  Series RLC Load/LConn1 -- Series RLC Load1/LConn1 -- Conn1/RConn1
  Series RLC Load2/RConn1 -- Conn5/RConn1
  IGBT/Diode/RConn1 -- E/RConn1
  Diode/RConn1 -- Current Measurement/LConn1 -- Series RLC Load2/LConn1
  Current Measurement/RConn1 -- Series RLC Load3/LConn1 -- Conn2/RConn1
  Series RLC Load3/RConn1 -- Conn6/RConn1
  Conn3/RConn1 -- Series RLC Load/RConn1

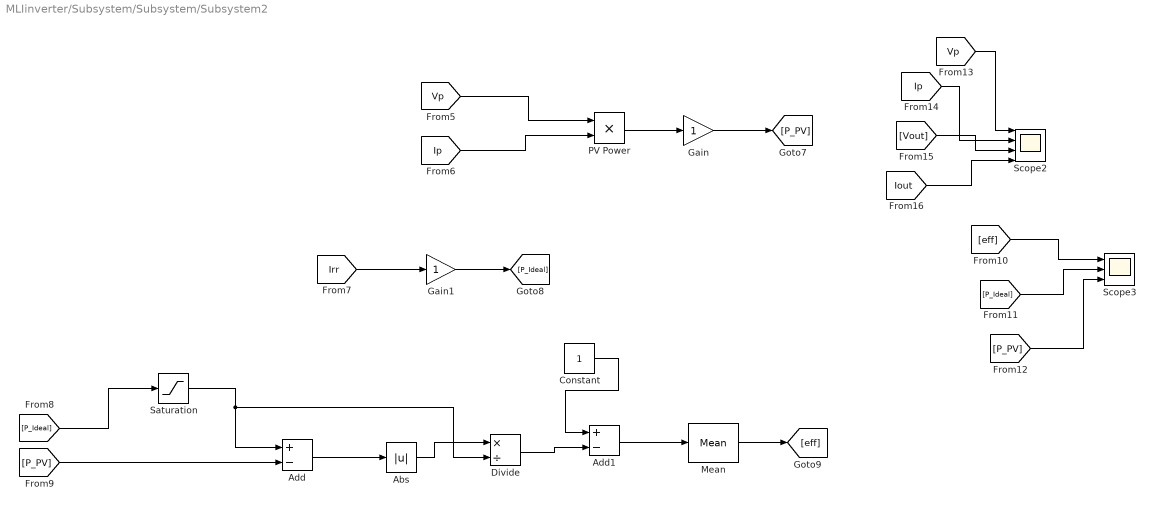
== system MLIinverter/Subsystem/Subsystem/Subsystem2 ==
  Abs : Abs
  Add : Sum  Inputs=+-
  Add1 : Sum  Inputs=+-
  Constant : Constant
  Divide : Product  Inputs=*/
  Gain : Gain
  Gain1 : Gain
  Mean : spsMeanLib/Mean  Freq=60  Vinit=0  Ts=0
  PV Power : Product
  Saturation : Saturate
  Scope2 : Scope  NumInputPorts=4
  Scope3 : Scope  NumInputPorts=3
  wires:
  [Irr] -> Gain1/1
  [Ip] -> PV Power/2
  Abs/1 -> Divide/1
  Add/1 -> Abs/1
  Mean/1 -> [eff]
  Constant/1 -> Add1/1
  PV Power/1 -> Gain/1
  Gain1/1 -> [P_Ideal]
  [Vp] -> PV Power/1
  [P_Ideal] -> Scope3/2
  Saturation/1 -> Divide/2, Add/1
  [P_PV] -> Scope3/3
  [eff] -> Scope3/1
  [P_Ideal] -> Saturation/1
  [Iout] -> Scope2/4
  [P_PV] -> Add/2
  [Vout] -> Scope2/3
  Gain/1 -> [P_PV]
  [Vp] -> Scope2/1
  Divide/1 -> Add1/2
  Add1/1 -> Mean/1
  [Ip] -> Scope2/2

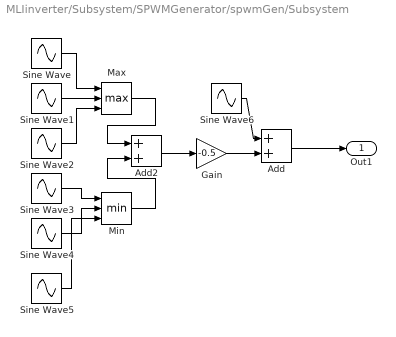
== system MLIinverter/Subsystem/SPWMGenerator/spwmGen/Subsystem ==
  Add : Sum
  Add2 : Sum
  Gain : Gain  Gain=-0.5
  Max : MinMax  Function=max  Inputs=3
  Min : MinMax  Inputs=3
  Sine Wave : Sin  Amplitude=2  Frequency=2*pi*50  SampleTime=0
  Sine Wave1 : Sin  Amplitude=2  Frequency=2*pi*50  Phase=2*pi/3  SampleTime=0
  Sine Wave2 : Sin  Amplitude=2  Frequency=2*pi*50  Phase=4*pi/3  SampleTime=0
  Sine Wave3 : Sin  Amplitude=2  Frequency=2*pi*50  SampleTime=0
  Sine Wave4 : Sin  Amplitude=2  Frequency=2*pi*50  Phase=2*pi/3  SampleTime=0
  Sine Wave5 : Sin  Amplitude=2  Frequency=2*pi*50  Phase=4*pi/3  SampleTime=0
  Sine Wave6 : Sin  Amplitude=2  Frequency=2*pi*50  SampleTime=0
  Out1 : Outport
  wires:
  Add/1 -> Out1/1
  Sine Wave4/1 -> Min/2
  Add2/1 -> Gain/1
  Sine Wave1/1 -> Max/2
  Sine Wave3/1 -> Min/1
  Sine Wave2/1 -> Max/3
  Max/1 -> Add2/1
  Min/1 -> Add2/2
  Sine Wave6/1 -> Add/1
  Sine Wave5/1 -> Min/3
  Gain/1 -> Add/2
  Sine Wave/1 -> Max/1

== system MLIinverter/Subsystem/SPWMGenerator/spwmGen1/Subsystem ==
  Add : Sum
  Add2 : Sum
  Gain : Gain  Gain=-0.5
  Max : MinMax  Function=max  Inputs=3
  Min : MinMax  Inputs=3
  Sine Wave : Sin  Amplitude=2  Frequency=2*pi*50  SampleTime=0
  Sine Wave1 : Sin  Amplitude=2  Frequency=2*pi*50  Phase=2*pi/3  SampleTime=0
  Sine Wave2 : Sin  Amplitude=2  Frequency=2*pi*50  Phase=4*pi/3  SampleTime=0
  Sine Wave3 : Sin  Amplitude=2  Frequency=2*pi*50  SampleTime=0
  Sine Wave4 : Sin  Amplitude=2  Frequency=2*pi*50  Phase=2*pi/3  SampleTime=0
  Sine Wave5 : Sin  Amplitude=2  Frequency=2*pi*50  Phase=4*pi/3  SampleTime=0
  Sine Wave6 : Sin  Amplitude=2  Frequency=2*pi*50  Phase=2*pi/3  SampleTime=0
  Out1 : Outport
  wires:
  Sine Wave5/1 -> Min/3
  Sine Wave3/1 -> Min/1
  Sine Wave1/1 -> Max/2
  Sine Wave/1 -> Max/1
  Min/1 -> Add2/2
  Max/1 -> Add2/1
  Sine Wave2/1 -> Max/3
  Sine Wave4/1 -> Min/2
  Add2/1 -> Gain/1
  Gain/1 -> Add/2
  Sine Wave6/1 -> Add/1
  Add/1 -> Out1/1

== system MLIinverter/Subsystem/SPWMGenerator/spwmGen2/Subsystem ==
  Add : Sum
  Add2 : Sum
  Gain : Gain  Gain=-0.5
  Max : MinMax  Function=max  Inputs=3
  Min : MinMax  Inputs=3
  Sine Wave : Sin  Amplitude=2  Frequency=2*pi*50  SampleTime=0
  Sine Wave1 : Sin  Amplitude=2  Frequency=2*pi*50  Phase=2*pi/3  SampleTime=0
  Sine Wave2 : Sin  Amplitude=2  Frequency=2*pi*50  Phase=4*pi/3  SampleTime=0
  Sine Wave3 : Sin  Amplitude=2  Frequency=2*pi*50  SampleTime=0
  Sine Wave4 : Sin  Amplitude=2  Frequency=2*pi*50  Phase=2*pi/3  SampleTime=0
  Sine Wave5 : Sin  Amplitude=2  Frequency=2*pi*50  Phase=4*pi/3  SampleTime=0
  Sine Wave6 : Sin  Amplitude=2  Frequency=2*pi*50  Phase=4*pi/3  SampleTime=0
  Out1 : Outport
  wires:
  Sine Wave5/1 -> Min/3
  Sine Wave3/1 -> Min/1
  Sine Wave1/1 -> Max/2
  Sine Wave/1 -> Max/1
  Min/1 -> Add2/2
  Max/1 -> Add2/1
  Sine Wave2/1 -> Max/3
  Sine Wave4/1 -> Min/2
  Add2/1 -> Gain/1
  Gain/1 -> Add/2
  Sine Wave6/1 -> Add/1
  Add/1 -> Out1/1

== system MLIinverter/Subsystem/Subsystem/Custom Neural Network/Layer 1 ==
  "p{1}" : Inport  PortDimensions=3
      mask Display: e = 0.06;c1 = [120 230 180]/255;c2 = ([120 230 180]+0)/(256+128);c3 = ([120 230 180]+128)/(256+128);patch([0 1 1 0],[0 0 1 1],c1);patch([0 1 1 1-e 1-e 0+e],[0 0 1 1-e 0+e 0+e],c2);patch([0 0 1 1-e 0+e 0+e],[0 1 1 1-e 1-e 0+e],c3);plot([0 1 1 0 0],[0 0 1 1 0]);
  Delays 1 : Subsystem
      mask Display: e = 0.06;c1 = [120 150 230]/255;c2 = ([120 150 230]+0)/383;c3 = ([120 150 230]+128)/383;patch([0 1 1 0],[0 0 1 1],c1);patch([0 1 1 1-e 1-e 0+e],[0 0 1 1-e 0+e 0+e],c2);patch([0 0 1 1-e 0+e 0+e],[0 1 1 1-e 1-e 0+e],c3);plot([0 1 1 0 0],[0 0 1 1 0]);disp('0');
  "IW{1,1}" : Subsystem
      mask Display: e = 0.06;c1 = [120 150 230]/255;c2 = ([120 150 230]+0)/383;c3 = ([120 150 230]+128)/383;patch([0 1 1 0],[0 0 1 1],c1);patch([0 1 1 1-e 1-e 0+e],[0 0 1 1-e 0+e 0+e],c2);patch([0 0 1 1-e 0+e 0+e],[0 1 1 1-e 1-e 0+e],c3);plot([0 1 1 0 0],[0 0 1 1 0]);disp('W');
  "b{1}" : Constant  Value=[6.0411307030171190746159481932409107685089111328125;-0.040993864256064292683756633550729020498692989349365234375;7.12165695142788290894486635806970298290252685546875]
      mask Display: e = 0.06;c1 = [120 150 230]/255;c2 = ([120 150 230]+0)/383;c3 = ([120 150 230]+128)/383;patch([0 1 1 0],[0 0 1 1],c1);patch([0 1 1 1-e 1-e 0+e],[0 0 1 1-e 0+e 0+e],c2);patch([0 0 1 1-e 0+e 0+e],[0 1 1 1-e 1-e 0+e],c3);plot([0 1 1 0 0],[0 0 1 1 0]);disp('b');
  logsig : neural/Transfer Functions/logsig
      settings: SourceProductBaseCode=NN
  netsum : Sum  Inputs=2  InputSameDT=on  SaturateOnIntegerOverflow=on  OutDataTypeStr=Inherit: Same as first input
      mask Display: e = 0.06;c1 = [120 150 230]/255;c2 = ([120 150 230]+0)/383;c3 = ([120 150 230]+128)/383;patch([0 1 1 0],[0 0 1 1],c1);patch([0 1 1 1-e 1-e 0+e],[0 0 1 1-e 0+e 0+e],c2);patch([0 0 1 1-e 0+e 0+e],[0 1 1 1-e 1-e 0+e],c3);plot([0 1 1 0 0],[0 0 1 1 0]);disp('+');
  "a{1}" : Outport  InitialOutput=[0;0;0]
      mask Display: e = 0.06;c1 = [120 230 180]/255;c2 = ([120 230 180]+0)/(256+128);c3 = ([120 230 180]+128)/(256+128);patch([0 1 1 0],[0 0 1 1],c1);patch([0 1 1 1-e 1-e 0+e],[0 0 1 1-e 0+e 0+e],c2);patch([0 0 1 1-e 0+e 0+e],[0 1 1 1-e 1-e 0+e],c3);plot([0 1 1 0 0],[0 0 1 1 0]);
  wires:
  "p{1}"/1 -> Delays 1/1("p{1}")
  Delays 1/1("pd{1,1}") -> "IW{1,1}"/1("pd{1,1}")
  "IW{1,1}"/1("iz{1,1}") -> netsum/1
  "b{1}"/1 -> netsum/2
  netsum/1 -> logsig/1
  logsig/1 -> "a{1}"/1

== system MLIinverter/Subsystem/Subsystem/Custom Neural Network/Layer 2 ==
  "a{1} " : Inport  PortDimensions=3
      mask Display: e = 0.06;c1 = [120 230 180]/255;c2 = ([120 230 180]+0)/(256+128);c3 = ([120 230 180]+128)/(256+128);patch([0 1 1 0],[0 0 1 1],c1);patch([0 1 1 1-e 1-e 0+e],[0 0 1 1-e 0+e 0+e],c2);patch([0 0 1 1-e 0+e 0+e],[0 1 1 1-e 1-e 0+e],c3);plot([0 1 1 0 0],[0 0 1 1 0]);
  Delays 1 : Subsystem
      mask Display: e = 0.06;c1 = [120 150 230]/255;c2 = ([120 150 230]+0)/383;c3 = ([120 150 230]+128)/383;patch([0 1 1 0],[0 0 1 1],c1);patch([0 1 1 1-e 1-e 0+e],[0 0 1 1-e 0+e 0+e],c2);patch([0 0 1 1-e 0+e 0+e],[0 1 1 1-e 1-e 0+e],c3);plot([0 1 1 0 0],[0 0 1 1 0]);disp('0');
  "LW{2,1}" : Subsystem
      mask Display: e = 0.06;c1 = [120 150 230]/255;c2 = ([120 150 230]+0)/383;c3 = ([120 150 230]+128)/383;patch([0 1 1 0],[0 0 1 1],c1);patch([0 1 1 1-e 1-e 0+e],[0 0 1 1-e 0+e 0+e],c2);patch([0 0 1 1-e 0+e 0+e],[0 1 1 1-e 1-e 0+e],c3);plot([0 1 1 0 0],[0 0 1 1 0]);disp('W');
  "b{2}" : Constant  Value=[7.451720629532051276555648655630648136138916015625;2.448358638692150091031862757517956197261810302734375;5.787020295138542991253416403196752071380615234375;-0.4795618159282846182378534649615176022052764892578125;4.1877845315932464842489935108460485935211181640625;0.8009444913895220619082238044939003884792327880859375;0.90859956300292943343066554007236845791339874267578125;-0.47357859284561698576254684667219407856464385986328125;0.376932593028165452420097381036612205207347869873046875;-5.6718091290293575212899668258614838123321533203125]
      mask Display: e = 0.06;c1 = [120 150 230]/255;c2 = ([120 150 230]+0)/383;c3 = ([120 150 230]+128)/383;patch([0 1 1 0],[0 0 1 1],c1);patch([0 1 1 1-e 1-e 0+e],[0 0 1 1-e 0+e 0+e],c2);patch([0 0 1 1-e 0+e 0+e],[0 1 1 1-e 1-e 0+e],c3);plot([0 1 1 0 0],[0 0 1 1 0]);disp('b');
  netsum : Sum  Inputs=2  InputSameDT=on  SaturateOnIntegerOverflow=on  OutDataTypeStr=Inherit: Same as first input
      mask Display: e = 0.06;c1 = [120 150 230]/255;c2 = ([120 150 230]+0)/383;c3 = ([120 150 230]+128)/383;patch([0 1 1 0],[0 0 1 1],c1);patch([0 1 1 1-e 1-e 0+e],[0 0 1 1-e 0+e 0+e],c2);patch([0 0 1 1-e 0+e 0+e],[0 1 1 1-e 1-e 0+e],c3);plot([0 1 1 0 0],[0 0 1 1 0]);disp('+');
  tansig : neural/Transfer Functions/tansig
  "a{2}" : Outport  InitialOutput=[0;0;0;0;0;0;0;0;0;0]
      mask Display: e = 0.06;c1 = [120 230 180]/255;c2 = ([120 230 180]+0)/(256+128);c3 = ([120 230 180]+128)/(256+128);patch([0 1 1 0],[0 0 1 1],c1);patch([0 1 1 1-e 1-e 0+e],[0 0 1 1-e 0+e 0+e],c2);patch([0 0 1 1-e 0+e 0+e],[0 1 1 1-e 1-e 0+e],c3);plot([0 1 1 0 0],[0 0 1 1 0]);
  wires:
  "a{1} "/1 -> Delays 1/1("p{2}")
  Delays 1/1("pd{2,1}") -> "LW{2,1}"/1("ad{2,1}")
  "LW{2,1}"/1("lz{2,1}") -> netsum/1
  "b{2}"/1 -> netsum/2
  netsum/1 -> tansig/1
  tansig/1 -> "a{2}"/1

== system MLIinverter/Subsystem/Subsystem/Custom Neural Network/Layer 3 ==
  "a{2} " : Inport  PortDimensions=10
      mask Display: e = 0.06;c1 = [120 230 180]/255;c2 = ([120 230 180]+0)/(256+128);c3 = ([120 230 180]+128)/(256+128);patch([0 1 1 0],[0 0 1 1],c1);patch([0 1 1 1-e 1-e 0+e],[0 0 1 1-e 0+e 0+e],c2);patch([0 0 1 1-e 0+e 0+e],[0 1 1 1-e 1-e 0+e],c3);plot([0 1 1 0 0],[0 0 1 1 0]);
  Delays 1 : Subsystem
      mask Display: e = 0.06;c1 = [120 150 230]/255;c2 = ([120 150 230]+0)/383;c3 = ([120 150 230]+128)/383;patch([0 1 1 0],[0 0 1 1],c1);patch([0 1 1 1-e 1-e 0+e],[0 0 1 1-e 0+e 0+e],c2);patch([0 0 1 1-e 0+e 0+e],[0 1 1 1-e 1-e 0+e],c3);plot([0 1 1 0 0],[0 0 1 1 0]);disp('0');
  "LW{3,2}" : Subsystem
      mask Display: e = 0.06;c1 = [120 150 230]/255;c2 = ([120 150 230]+0)/383;c3 = ([120 150 230]+128)/383;patch([0 1 1 0],[0 0 1 1],c1);patch([0 1 1 1-e 1-e 0+e],[0 0 1 1-e 0+e 0+e],c2);patch([0 0 1 1-e 0+e 0+e],[0 1 1 1-e 1-e 0+e],c3);plot([0 1 1 0 0],[0 0 1 1 0]);disp('W');
  "b{3}" : Constant  Value=-0.70129746558378958098955990863032639026641845703125
      mask Display: e = 0.06;c1 = [120 150 230]/255;c2 = ([120 150 230]+0)/383;c3 = ([120 150 230]+128)/383;patch([0 1 1 0],[0 0 1 1],c1);patch([0 1 1 1-e 1-e 0+e],[0 0 1 1-e 0+e 0+e],c2);patch([0 0 1 1-e 0+e 0+e],[0 1 1 1-e 1-e 0+e],c3);plot([0 1 1 0 0],[0 0 1 1 0]);disp('b');
  netsum : Sum  Inputs=2  InputSameDT=on  SaturateOnIntegerOverflow=on  OutDataTypeStr=Inherit: Same as first input
      mask Display: e = 0.06;c1 = [120 150 230]/255;c2 = ([120 150 230]+0)/383;c3 = ([120 150 230]+128)/383;patch([0 1 1 0],[0 0 1 1],c1);patch([0 1 1 1-e 1-e 0+e],[0 0 1 1-e 0+e 0+e],c2);patch([0 0 1 1-e 0+e 0+e],[0 1 1 1-e 1-e 0+e],c3);plot([0 1 1 0 0],[0 0 1 1 0]);disp('+');
  tansig : neural/Transfer Functions/tansig
  "a{3}" : Outport  InitialOutput=0
      mask Display: e = 0.06;c1 = [120 230 180]/255;c2 = ([120 230 180]+0)/(256+128);c3 = ([120 230 180]+128)/(256+128);patch([0 1 1 0],[0 0 1 1],c1);patch([0 1 1 1-e 1-e 0+e],[0 0 1 1-e 0+e 0+e],c2);patch([0 0 1 1-e 0+e 0+e],[0 1 1 1-e 1-e 0+e],c3);plot([0 1 1 0 0],[0 0 1 1 0]);
  wires:
  "a{2} "/1 -> Delays 1/1("p{3}")
  Delays 1/1("pd{3,2}") -> "LW{3,2}"/1("ad{3,2}")
  "LW{3,2}"/1("lz{3,2}") -> netsum/1
  "b{3}"/1 -> netsum/2
  netsum/1 -> tansig/1
  tansig/1 -> "a{3}"/1

== system MLIinverter/Subsystem/Subsystem/Custom Neural Network/Process Input 1 ==
  x : Inport  PortDimensions=3
      mask Display: e = 0.06;c1 = [120 230 180]/255;c2 = ([120 230 180]+0)/(256+128);c3 = ([120 230 180]+128)/(256+128);patch([0 1 1 0],[0 0 1 1],c1);patch([0 1 1 1-e 1-e 0+e],[0 0 1 1-e 0+e 0+e],c2);patch([0 0 1 1-e 0+e 0+e],[0 1 1 1-e 1-e 0+e],c3);plot([0 1 1 0 0],[0 0 1 1 0]);
  mapminmax : neural/Processing Functions/mapminmax  xmin=[0;0;12.3692438683199998905593020027]  xmax=[998.207477106809051292657386512;16.9750000000000014210854715202;15.452546757560300605405245733]  ymin=-1  ymax=1
  p : Outport  PortDimensions=3
      mask Display: e = 0.06;c1 = [120 230 180]/255;c2 = ([120 230 180]+0)/(256+128);c3 = ([120 230 180]+128)/(256+128);patch([0 1 1 0],[0 0 1 1],c1);patch([0 1 1 1-e 1-e 0+e],[0 0 1 1-e 0+e 0+e],c2);patch([0 0 1 1-e 0+e 0+e],[0 1 1 1-e 1-e 0+e],c3);plot([0 1 1 0 0],[0 0 1 1 0]);
  wires:
  x/1 -> mapminmax/1
  mapminmax/1 -> p/1

== system MLIinverter/Subsystem/Subsystem/Custom Neural Network/Process Output 1 ==
  a : Inport  PortDimensions=1
      mask Display: e = 0.06;c1 = [120 230 180]/255;c2 = ([120 230 180]+0)/(256+128);c3 = ([120 230 180]+128)/(256+128);patch([0 1 1 0],[0 0 1 1],c1);patch([0 1 1 1-e 1-e 0+e],[0 0 1 1-e 0+e 0+e],c2);patch([0 0 1 1-e 0+e 0+e],[0 1 1 1-e 1-e 0+e],c3);plot([0 1 1 0 0],[0 0 1 1 0]);
  mapminmax_reverse : neural/Processing Functions/mapminmax_reverse  xmin=113.797726374902993029536446556  xmax=142.164283155253997392719611526  ymin=-1  ymax=1
  y : Outport  PortDimensions=1
      mask Display: e = 0.06;c1 = [120 230 180]/255;c2 = ([120 230 180]+0)/(256+128);c3 = ([120 230 180]+128)/(256+128);patch([0 1 1 0],[0 0 1 1],c1);patch([0 1 1 1-e 1-e 0+e],[0 0 1 1-e 0+e 0+e],c2);patch([0 0 1 1-e 0+e 0+e],[0 1 1 1-e 1-e 0+e],c3);plot([0 1 1 0 0],[0 0 1 1 0]);
  wires:
  a/1 -> mapminmax_reverse/1
  mapminmax_reverse/1 -> y/1

== system MLIinverter/Subsystem/Subsystem/Subsystem1/Subsystem ==
  In1 : Inport
  In2 : Inport  Port=2
  Add : Sum
  Add1 : Sum
  Constant : Constant  Value=0.56
  Dead Zone : DeadZone  SaturateOnIntegerOverflow=on
  Discrete PID Controller : pid_lib/PID Controller  Controller=PID  Form=Parallel  TimeDomain=Discrete-time  UseExternalTs=off  SampleTime=-1  IntegratorMethod=Forward Euler  FilterMethod=Forward Euler  ControllerParametersSource=internal  P=1  I=1  D=0  UseFilter=on  N=100  TunerSelectOption=Transfer Function Based (PID Tuner App)  InitialConditionSource=internal  InitialConditionForIntegrator=0  InitialConditionForFilter=0  DifferentiatorICPrevScaledInput=0  ExternalReset=none  TrackingMode=off  Kt=1  LimitOutput=off  SatLimitsSource=internal  UpperSaturationLimit=inf  LowerSaturationLimit=-inf  LinearizeAsGain=off  AntiWindupMode=none  Kb=1  POutMin=[]  POutMax=[]  IOutMin=[]  IOutMax=[]  DOutMin=[]  DOutMax=[]  NOutMin=[]  NOutMax=[]  SumOutMin=[]  SumOutMax=[]  SaturationOutMin=[]  SaturationOutMax=[]  PParamMin=[]  PParamMax=[]  IParamMin=[]  IParamMax=[]  DParamMin=[]  DParamMax=[]  NParamMin=[]  NParamMax=[]  KbParamMin=[]  KbParamMax=[]  KtParamMin=[]  KtParamMax=[]  KbOutMin=[]  KbOutMax=[]  KtOutMin=[]  KtOutMax=[]  IntegratorOutMin=[]  IntegratorOutMax=[]  FilterOutMin=[]  FilterOutMax=[]  SumI1OutMin=[]  SumI1OutMax=[]  SumI2OutMin=[]  SumI2OutMax=[]  SumI3OutMin=[]  SumI3OutMax=[]  SumI4OutMin=[]  SumI4OutMax=[]  SumDOutMin=[]  SumDOutMax=[]  DifferentiatorOutMin=[]  DifferentiatorOutMax=[]  FilterDiffOutCoefMin=[]  FilterDiffOutCoefMax=[]  ReciprocalOutMin=[]  ReciprocalOutMax=[]  SumDenOutMin=[]  SumDenOutMax=[]  SumNumOutMin=[]  SumNumOutMax=[]  DivideOutMin=[]  DivideOutMax=[]  UdiffTsProdOutMin=[]  UdiffTsProdOutMax=[]  NTsProdOutMin=[]  NTsProdOutMax=[]  UintegralTsProdOutMin=[]  UintegralTsProdOutMax=[]  UngainTsProdOutMin=[]  UngainTsProdOutMax=[]  IntegratorContinuousStateAttributes=''  IntegratorStateMustResolveToSignalObject=off  IntegratorRTWStateStorageClass=Auto  FilterContinuousStateAttributes=''  FilterStateMustResolveToSignalObject=off  FilterRTWStateStorageClass=Auto  ParallelPVariant=InternalParameters  IdealPVariant=Disabled  IVariant=InternalParameters  DVariant=InternalParameters  IntegratorVariant=Discrete  SatVariant=Disabled  AWVariant=Passthrough  PCopyVariant=Disabled  TRVariant=Disabled  FdbkBlocksVariant=Forward  IdealPFdbkVariant=Disabled  SatFdbkVariant=Disabled  DerivativeFilterVariant=ForwardEulerFilter  NVariant=InternalParameters  NCopyVariant=Disabled  FilterICVariant=InternalICsFilter  IntegratorICVariant=InternalICs  ExternalResetVariant=Disabled  TRSumVariant=Passthrough  SumFdbkVariant=Disabled  SumVariant=Sum_PID  TsampFilterVariant=InternalTs  TsampNgainVariant=Passthrough  TsampIntegralVariant=Passthrough  ExternalSaturationOutDataTypeStr=Inherit: Same as second input
  PWM Generator (DC-DC) : spsPWMGeneratorDCDCLib/PWM Generator (DC-DC)  Fsw=5000  Ts=0
  Saturation : Saturate
  Out1 : Outport  Description=""
  wires:
  In1/1 -> Add/2
  In2/1 -> Add/1
  Dead Zone/1 -> Discrete PID Controller/1
  Constant/1 -> Add1/1
  Add1/1 -> Saturation/1
  Discrete PID Controller/1 -> Add1/2
  Add/1 -> Dead Zone/1
  Saturation/1 -> PWM Generator (DC-DC)/1
  PWM Generator (DC-DC)/1 -> Out1/1

== system MLIinverter/Subsystem/Subsystem/Custom Neural Network/Layer 1/Delays 1 ==
  "p{1}" : Inport  PortDimensions=3
      mask Display: e = 0.06;c1 = [120 230 180]/255;c2 = ([120 230 180]+0)/(256+128);c3 = ([120 230 180]+128)/(256+128);patch([0 1 1 0],[0 0 1 1],c1);patch([0 1 1 1-e 1-e 0+e],[0 0 1 1-e 0+e 0+e],c2);patch([0 0 1 1-e 0+e 0+e],[0 1 1 1-e 1-e 0+e],c3);plot([0 1 1 0 0],[0 0 1 1 0]);
  mux : Mux  Inputs=1
      mask Display: e = 0.06;c1 = [120 150 230]/255;c2 = ([120 150 230]+0)/383;c3 = ([120 150 230]+128)/383;patch([0 1 1 0],[0 0 1 1],c1);patch([0 1 1 1-e 1-e 0+e],[0 0 1 1-e 0+e 0+e],c2);patch([0 0 1 1-e 0+e 0+e],[0 1 1 1-e 1-e 0+e],c3);plot([0 1 1 0 0],[0 0 1 1 0]);disp('Mux')
  "pd{1,1}" : Outport
      mask Display: e = 0.06;c1 = [120 230 180]/255;c2 = ([120 230 180]+0)/(256+128);c3 = ([120 230 180]+128)/(256+128);patch([0 1 1 0],[0 0 1 1],c1);patch([0 1 1 1-e 1-e 0+e],[0 0 1 1-e 0+e 0+e],c2);patch([0 0 1 1-e 0+e 0+e],[0 1 1 1-e 1-e 0+e],c3);plot([0 1 1 0 0],[0 0 1 1 0]);
  wires:
  "p{1}"/1 -> mux/1
  mux/1 -> "pd{1,1}"/1
